simulink model "dc5_example"  (R2019a)
settings: Solver=FixedStepDiscrete  StartTime=0.0  StopTime=4  RelTol=1e-3  EnableMultiTasking=on
PreLoadFcn:
  | Ts=1e-6;
libraries: powerlib x4, electricdrivelib x1, powerlib_meascontrol x1
Description:
  | Copyright 2008-2019 The MathWorks, Inc.
settings Model: ExtModeAutoUpdateStatusClock=off  Creator=MathWorks  LastModifiedBy=Phong
settings DataIOCC: LimitDataPoints=on  SaveFormat=Array  SignalLoggingSaveFormat=ModelDataLogs  SaveOutput=off  SignalLogging=off  SaveTime=off  ReturnWorkspaceOutputs=off  SignalLoggingName=sigsOut
settings OptimizationCC: ExpressionDepthLimit=2147483647  InitFltsAndDblsToZero=on  LifeSpan=inf
settings DebuggingCC: UnderspecifiedInitializationDetection=Classic  MergeDetectMultiDrivingBlocksExec=none  CheckExecutionContextPreStartOutputMsg=on  CheckExecutionContextRuntimeOutputMsg=on  SignalResolutionControl=TryResolveAllWithWarning  MultiTaskDSMMsg=warning  MultiTaskCondExecSysMsg=none  FcnCallInpInsideContextMsg=warning  StateNameClashWarn=warning  SFUnexpectedBacktrackingDiag=warning  SFNoUnconditionalDefaultTransitionDiag=warning  SFExecutionAtInitializationDiag=none  ArithmeticOperatorsInVariantConditions=warning
settings HardwareCC: ProdBitPerPointer=32  ProdBitPerSizeT=32  ProdBitPerPtrDiffT=32  ProdLargestAtomicFloat=None  ProdIntDivRoundTo=Undefined  ProdEndianess=Unspecified  ProdWordSize=32  ProdHWDeviceType=32-bit Generic  TargetUnknown=on
settings ModelReferenceCC: PropagateSignalLabelsOutOfModel=off
settings SFSimCC: SimUseLocalCustomCode=off
settings RTWCC: RTWUseLocalCustomCode=off
settings CodeAppCC: StateflowObjectComments=on
settings GRTTargetCC: TargetLangStandard=C89/C90 (ANSI)  GeneratePreprocessorConditionals=Disable all  CombineOutputUpdateFcns=off  GRTInterface=on
settings ConfigComp: CovMetricSettings=dw  CovHtmlReporting=on  CovSaveCumulativeToWorkspaceVar=on  CovSaveSingleToWorkspaceVar=on  CovExternalEMLEnable=off  CovSFcnEnable=off
settings SimscapeCC: SimscapeNormalizeSystem=off

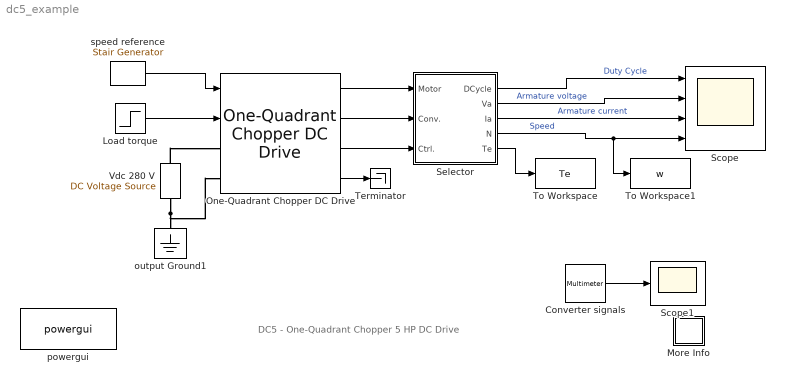
== system dc5_example ==
  note: DC5 - One-Quadrant Chopper 5 HP DC Drive
  Converter signals : powerlib/Measurements/Multimeter  PhasorSimulation=off  OutputType=Complex  sel=1  L=5  Gain=0  yselected={}  PSBOutputType=1  PSBequivalent=0  AxesSetting=[0,0.1,-100,100]  Display=0  SavedBlockNames=-11
      settings: SourceProductName=Simscape Electrical
  Load torque : Step  Time=2.5  Before=15  After=20  SampleTime=0
  More Info : Subsystem
      settings: OpenFcn=showdemo(bdroot(gcb))
      mask Display: disp('?')
  One-Quadrant Chopper DC Drive : electricdrivelib/DC drives/One-Quadrant Chopper DC Drive  Laf=1.234  Ra=0.78  La=0.016  Rf=150  Lf=112.5  J=0.25  Bm=0.01  Tfriction=0  w0=0  smoothingInductance=10e-3  Vfield=150  Ron=1e-3  Vf=1.3  Tf=0  Tt=0  Vfd=1.3  Rsnb=10e3  Csnb=inf  regulationType=Speed regulation  wb=1750  InitialSpeed=0  fc_sc=40  Tsc=100e-6  kp_sc=Kpw  ki_sc=Kiw  Acc=250  Dec=-250  fc_ic=500  refLim=1.5  switchfreq=5e3  Tic=20e-6  Pb=5*746  Vb=240  kp_ic=Kpi  ki_ic=Kii  baseSampleTime=5e-05  outputBusMode=Multiple output buses  busLabels=off  MechanicalLoad=Torque Tm  modelDetailLevel=Detailed  driveType=DC5  AverageValue=off
      settings: SourceProductName=Simscape Electrical  SourceProductBaseCode=PS
  Scope : Scope  NumInputPorts=4
  Scope1 : Scope
  Selector : Subsystem
  Terminator : Terminator
  To Workspace : ToWorkspace  VariableName=Te  SampleTime=-1
      settings: Save2DSignal=2-D array (concatenate along first dimension)
  To Workspace1 : ToWorkspace  VariableName=w  SampleTime=-1
      settings: Save2DSignal=2-D array (concatenate along first dimension)
  "Vdc 280 V " : powerlib/Electrical Sources/DC Voltage Source  Description=source block  Amplitude=280  Measurements=None
      settings: AttributesFormatString=\n  SourceProductName=Simscape Electrical
  output Ground1 : powerlib/Elements/Ground  LConnTagsString=a
      settings: SourceProductName=Simscape Electrical
  powergui : powerlib/powergui  Priority=2  SimulationMode=Discrete  SampleTime=Ts  frequency=60  Iterations=50  frequencyindice=0  Pbase=100e6  ErrMax=1e-4  UnitsV=kV  UnitsW=MW  buscounter=0  FunctionMessages=off  echomessages=off  EnableUseOfTLC=off  CurrentSourceSwitches=off  DisableSnubberDevices=off  DisableRonSwitches=off  DisableVfSwitches=off  DisplayEquations=off  AutomaticDiscreteSolvers=off  SolverType=Tustin/Backward Euler (TBE)  Interpol=off  ExternalGateDelay=off  methode=off  Ts=0  x0status=blocks  SPID=off  SwTol=0  HookPort=off  NonlinearTolerance=0  nMaxIteration=15  ContinueOnMaxIteration=off  RestoreLinks=warning  ResistiveCurrentMeasurement=off  Frange=[0:2:500]  Ylog=off  Xlog=on  ShowGrid=off  save=off  variable=ZData  structure=0  ZoomFFT=on  StartTime=0.0  cycles=1  DisplayStyle=1  fundamental=60  FreqAxis=off  MaxFrequency=1000  frequencyindicesteady=1  RmsSteady=1  display=off
      settings: SourceProductName=Simscape Electrical
  speed reference : powerlib_meascontrol/Pulse & Signal Generators/Stair Generator  t=[0.05 2 3]  e=[100 200 150]  Ts=Ts
      settings: SourceProductName=Simscape Electrical
  wires:
  One-Quadrant Chopper DC Drive/1 -> Selector/1(Motor)
  One-Quadrant Chopper DC Drive/2 -> Selector/2(Conv.)
  One-Quadrant Chopper DC Drive/3 -> Selector/3(Ctrl.)
  speed reference/1 -> One-Quadrant Chopper DC Drive/1
  Load torque/1 -> One-Quadrant Chopper DC Drive/2
  Converter signals/1 -> Scope1/1
  Selector/1(DCycle) -> Scope/1  "Duty Cycle"
  Selector/2(Va) -> Scope/2  "Armature voltage"
  Selector/3(Ia) -> Scope/3  "Armature current"
  Selector/4(N) -> Scope/4, To Workspace1/1  "Speed"
  One-Quadrant Chopper DC Drive/4 -> Terminator/1
  Selector/5(Te) -> To Workspace/1
  connections:
  "Vdc 280 V "/RConn1 -- One-Quadrant Chopper DC Drive/LConn1
  "Vdc 280 V "/LConn1 -- One-Quadrant Chopper DC Drive/LConn2 -- output Ground1/LConn1

== system dc5_example/More Info ==

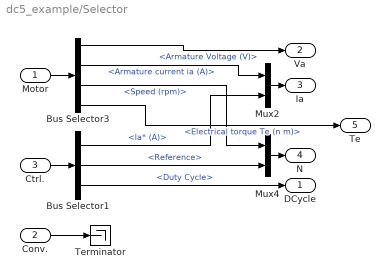
== system dc5_example/Selector ==
  Motor : Inport
  Conv. : Inport  Port=2
  Ctrl. : Inport  Port=3
  Bus Selector1 : BusSelector  OutputSignals=Ia* (A),Reference,Duty Cycle
  Bus Selector3 : BusSelector  OutputSignals=Armature Voltage (V),Armature current ia (A),Speed (rpm),Electrical torque Te (n m)
  Mux2 : Mux  Inputs=2
  Mux4 : Mux  Inputs=2
  Terminator : Terminator
  DCycle : Outport
  Va : Outport  Port=2
  Ia : Outport  Port=3
  N : Outport  Port=4
  Te : Outport  Port=5
  wires:
  Mux2/1 -> Ia/1
  Mux4/1 -> N/1
  Motor/1 -> Bus Selector3/1
  Bus Selector3/1 -> Va/1  "<Armature Voltage (V)>"
  Ctrl./1 -> Bus Selector1/1
  Bus Selector1/1 -> Mux2/2  "<Ia* (A)>"
  Bus Selector1/2 -> Mux4/2  "<Reference>"
  Bus Selector3/2 -> Mux2/1  "<Armature current ia (A)>"
  Bus Selector3/3 -> Mux4/1  "<Speed (rpm)>"
  Conv./1 -> Terminator/1
  Bus Selector1/3 -> DCycle/1  "<Duty Cycle>"
  Bus Selector3/4 -> Te/1  "<Electrical torque Te (n m)>"
